simulink model "Car_model"  (R2021b)
settings: Solver=VariableStepAuto  StartTime=0.0  StopTime=8  RelTol=1e-3
libraries: simulink x1, fuzblock x1
settings Model: Creator=E Club  LastModifiedBy=E Club

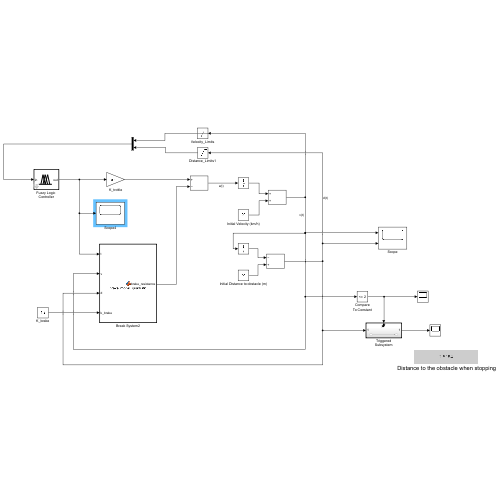
[thumbnail: Simulink's stored preview of the top-level diagram]
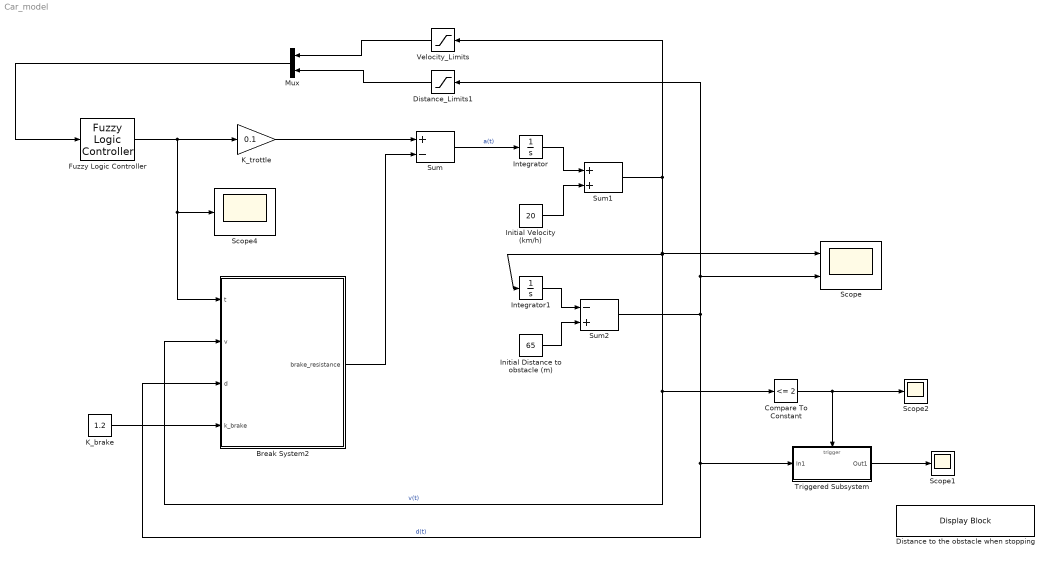
== system Car_model ==
  " Distance to the obstacle when stopping" : DisplayBlock  LabelPosition=Hide  Format=short  Transparency=1
  Break System2 : MATLAB Function  TreatAsAtomicUnit=on
  Compare To Constant : simulink/Logic and Bit Operations/Compare To Constant  relop=<=  const=2  OutDataTypeStr=boolean
  Distance_Limits1 : Saturate  UpperLimit=80  LowerLimit=0
  Fuzzy Logic Controller : fuzblock/Fuzzy Logic  Controller  FIS='FLC_collsion_avoidance.fis'  OutputSampleNumber=101  DataType=single  FuzzifiedInputs=off  RuleFiringStrengths=off  RuleOutputs=off  AggregatedOutputs=off  SimulateUsing=Interpreted execution  OutOfRangeInputValueMessage=warning  NoRuleFiredMessage=warning  EmptyOutputFuzzySetMessage=warning
  Initial Distance to obstacle (m) : Constant  Value=65
  Initial Velocity (km/h) : Constant  Value=20
  Integrator : Integrator
  Integrator1 : Integrator
  K_brake : Constant  Value=1.2
  K_trottle : Gain  Gain=0.1
  Mux : Mux  Inputs=2
  Scope : Scope  NumInputPorts=2
  Scope1 : Scope
  Scope2 : Scope
  Scope4 : Scope
  Sum : Sum  Inputs=+-
  Sum1 : Sum
  Sum2 : Sum  Inputs=-+
  Triggered Subsystem : Subsystem  TreatAsAtomicUnit=on
  Velocity_Limits : Saturate  UpperLimit=180  LowerLimit=0
  wires:
  Fuzzy Logic Controller/1 -> Break System2/1(t), Scope4/1, K_trottle/1
  K_trottle/1 -> Sum/1
  Break System2/1(brake_resistance) -> Sum/2
  Sum/1 -> Integrator/1  "a(t)"
  Integrator/1 -> Sum1/1
  Initial Velocity (km/h)/1 -> Sum1/2
  Sum1/1 -> Velocity_Limits/1, Break System2/2(v), Compare To Constant/1, Integrator1/1, Scope/1  "v(t)"
  Integrator1/1 -> Sum2/1
  Initial Distance to obstacle (m)/1 -> Sum2/2
  Sum2/1 -> Scope/2, Distance_Limits1/1, Break System2/3(d), Triggered Subsystem/1(In1)  "d(t)"
  Velocity_Limits/1 -> Mux/1
  Distance_Limits1/1 -> Mux/2
  Mux/1 -> Fuzzy Logic Controller/1
  K_brake/1 -> Break System2/4(k_brake)
  Compare To Constant/1 -> Scope2/1, Triggered Subsystem/Trigger
  Triggered Subsystem/1(Out1) -> Scope1/1

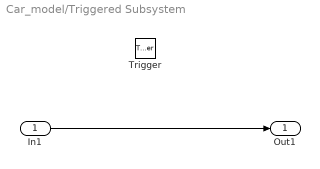
== system Car_model/Triggered Subsystem ==
  In1 : Inport
  Trigger : TriggerPort  VariantControl=(inherit)
  Out1 : Outport
  wires:
  In1/1 -> Out1/1

== matlab function Car_model/Break System2 ==
  data: t input; brake_resistance output; v input; d input; k_brake input
function brake_resistance = brake_model_quadratic(t, v, d, k_brake)
    d = max(d, 0.1);  % Prevent division by zero
    brake_resistance = k_brake * v^2 / d;
  
end
